simulink model "sraPrac2"  (R2025b)
settings: Solver=FixedStepAuto  StartTime=0.0  StopTime=2  RelTol=1e-3
settings Model: Creator=Entrar  LastModifiedBy=lily

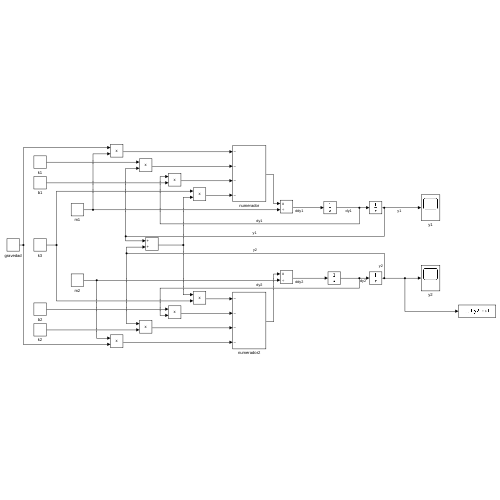
[thumbnail: Simulink's stored preview of the top-level diagram]
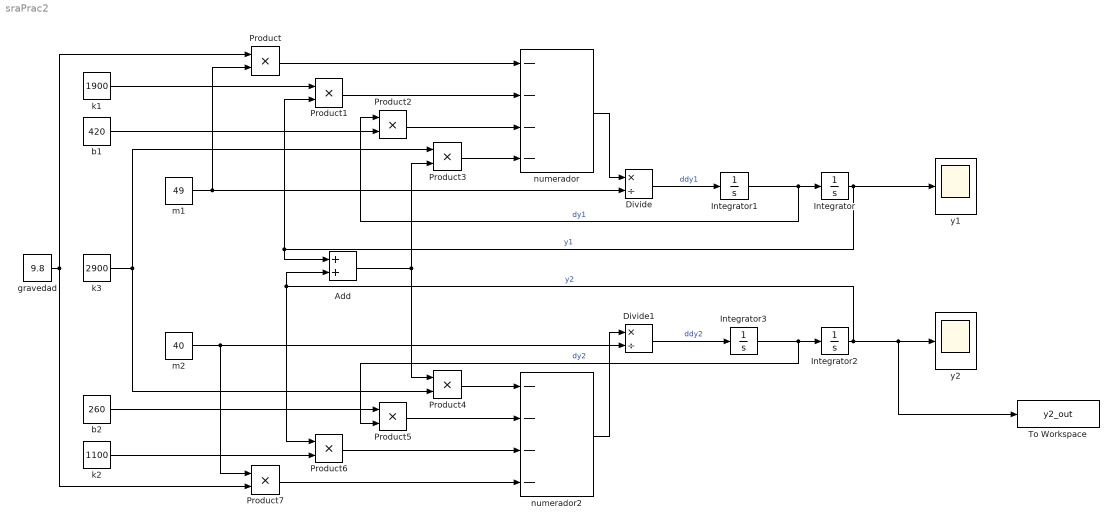
== system sraPrac2 ==
  Add : Sum
  Divide : Product  Inputs=*/
  Divide1 : Product  Inputs=*/
  Integrator{,1..3} (4 alike) : Integrator
  Product{,1..7} (8 alike) : Product
  To Workspace : ToWorkspace  VariableName=y2_out  SampleTime=-1
      settings: Save2DSignal=2-D array (concatenate along first dimension)
  b1 : Constant  Value=420
  b2 : Constant  Value=260
  gravedad : Constant  Value=9.8
  k1 : Constant  Value=1900
  k2 : Constant  Value=1100
  k3 : Constant  Value=2900
  m1 : Constant  Value=49
  m2 : Constant  Value=40
  numerador : Sum  Inputs=----
  numerador2 : Sum  Inputs=----
  y1 : Scope
      settings: Description=y  ActiveDisplayYMinimum=-1  ActiveDisplayYMaximum=1
  y2 : Scope
      settings: Description=y  ActiveDisplayYMinimum=-0.09363810954148484  ActiveDisplayYMaximum=0.010404234393498314
  wires:
  Integrator1/1 -> Product2/1, Integrator/1  "dy1"
  gravedad/1 -> Product/1, Product7/2
  m1/1 -> Product/2, Divide/2
  Product/1 -> numerador/1
  Integrator/1 -> y1/1, Add/1, Product1/2  "y1"
  Divide/1 -> Integrator1/1  "ddy1"
  numerador/1 -> Divide/1
  k1/1 -> Product1/1
  Product1/1 -> numerador/2
  b1/1 -> Product2/2
  Product2/1 -> numerador/3
  Integrator3/1 -> Product5/2, Integrator2/1  "dy2"
  Integrator2/1 -> Product6/1, Add/2, To Workspace/1, y2/1  "y2"
  Add/1 -> Product4/1, Product3/2
  k3/1 -> Product3/1, Product4/2
  Product3/1 -> numerador/4
  Divide1/1 -> Integrator3/1  "ddy2"
  numerador2/1 -> Divide1/1
  Product4/1 -> numerador2/1
  b2/1 -> Product5/1
  Product5/1 -> numerador2/2
  k2/1 -> Product6/2
  Product6/1 -> numerador2/3
  m2/1 -> Product7/1, Divide1/2
  Product7/1 -> numerador2/4
